simulink model "embedded_func_in_cond"  (Simulink 7.6)
settings: Solver=FixedStepDiscrete  StartTime=0.0  StopTime=10.0  FixedStep=1  RelTol=1e-3
settings Model: Creator=Harmon S. Nine  LastModifiedBy=c2wt
settings DebuggingCC: StrictBusMsg=Warning
settings SFSimCC: SimParseCustomCode=off

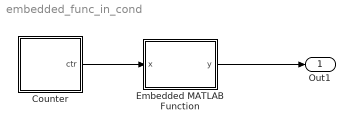
== system embedded_func_in_cond ==
  Counter : Stateflow chart  TreatAsAtomicUnit=on
  Embedded MATLAB Function : Stateflow chart  TreatAsAtomicUnit=on
  Out1 : Outport
  wires:
  Embedded MATLAB Function/1(y) -> Out1/1
  Counter/1(ctr) -> Embedded MATLAB Function/1(x)

== stateflow chart Counter ==
  state s1
  (default) -> s1
  s1 -> s1 [order 1] : [ctr < 10] / ctr = ctr+1;
  s1 -> s1 [order 2] : [ctr >= 10 ] / ctr = 0;
  data: ctr output double =1

== matlab function Embedded MATLAB Function ==
  data: y output double; x input double
function y = fcn( x )
%#eml

if isone( x )
  y = -1
elseif istwo( x )
  y = -2
elseif isthree( x )
  y = -3
elseif x == 4
  y = -4
elseif isfive( x )
  y = -5
elseif x == 6
  y = -6
elseif x == 7
  y = -7
elseif iseight( x )
  y = -8
else
  y = x
end
